simulink model "metro_queue"  (R2018b)
settings: Solver=VariableStepAuto  StartTime=0.0  StopTime=10.0  RelTol=1e-3
values from neighbouring files (symbols this model uses):
  entity_gen_period = 1.0 / current_mean_intensity    [metro_script.m]
undefined symbols (not defined in the file or in its folder): des
libraries: simeventslib x2
settings Model: Creator=kotvo  LastModifiedBy=marky

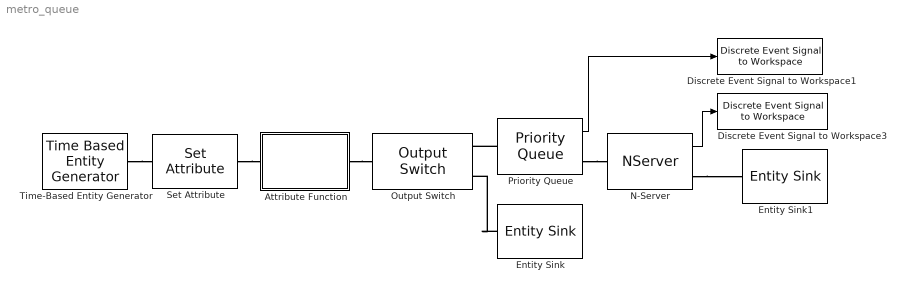
== system metro_queue ==
  Attribute Function : Subsystem  LoadFcn=des.afb.attributefunction_support(gcb,'LoadFcn');  StartFcn=des.afb.attributefunction_support(gcb,'StartFcn');  mask(Attribute Function){OutputNamePrefix=out_}
      mask prompts: OutputNamePrefix "Prefix name"
      settings: CopyFcn=des.afb.attributefunction_support(gcb,'CopyFcn');  OpenFcn=des.afb.attributefunction_support(gcb,'OpenFcn');  ErrorFcn=des.afb.error_redirect
      mask Help: slhelp(gcbh)
      mask Display: image(des_iconLoad('attribFunction.jpg'),'center');
  Discrete Event Signal to Workspace1 : simeventslib/SimEvents Sinks/Discrete Event Signal to Workspace  VariableName=average_wait  SaveFormat=Array  isMonitorOnly=off  isRecordIC=off
      settings: SourceProductName=SimEvents  SourceProductBaseCode=SE
  Discrete Event Signal to Workspace3 : simeventslib/SimEvents Sinks/Discrete Event Signal to Workspace  VariableName=processed_requests  SaveFormat=Array  isMonitorOnly=off  isRecordIC=off
      settings: SourceProductName=SimEvents  SourceProductBaseCode=SE
  Entity Sink : EntitySink
  Entity Sink1 : EntitySink
  N-Server : NServer  NumberOfServers=3  ServiceTime=2  StatNumberDeparted=on
  Output Switch : OutputSwitch  NumberOutputPorts=2
  Priority Queue : PriorityQueue  Capacity=current_queue_capacity  SortingAttributeName=priority  StatAverageWait=on
      settings: OutputPortMap=o2
  Set Attribute : SetAttribute  AttributeName=priority  EvaluatedAttributeValue={ 1}
  Time-Based Entity Generator : TimeBasedEntityGenerator  Distribution=Exponential  Period=entity_gen_period  Maximum=5  Mean=entity_gen_period
  wires:
  N-Server/1 -> Discrete Event Signal to Workspace3/1
  Priority Queue/1 -> Discrete Event Signal to Workspace1/1
  connections:
  Entity Sink/LConn1 -- Output Switch/RConn2
  Priority Queue/LConn1 -- Output Switch/RConn1
  N-Server/RConn1 -- Entity Sink1/LConn1
  Set Attribute/RConn1 -- Attribute Function/LConn1
  Attribute Function/RConn1 -- Output Switch/LConn1
  Priority Queue/RConn1 -- N-Server/LConn1
  Time-Based Entity Generator/RConn1 -- Set Attribute/LConn1

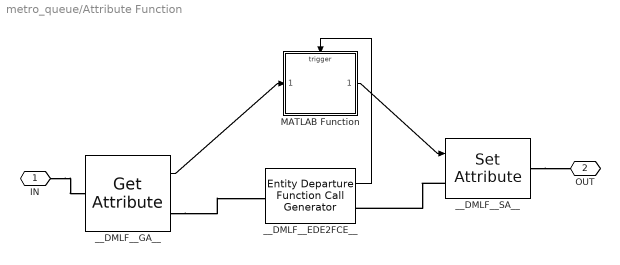
== system metro_queue/Attribute Function ==
  MATLAB Function : MATLAB Function  TreatAsAtomicUnit=on
  __DMLF__EDE2FCE__ : EntityDepartureFunctionCallGenerator  TimingFunctionCallF1=Before entity departure  IsInsideAFB=on
  __DMLF__GA__ : GetAttribute  AttributeName=priority  AttributeSendTiming=Before entity departure  EvaluatedDefaultAttributeValue={ []}  IsInsideAFB=on
      settings: OutputPortMap=o1
  __DMLF__SA__ : SetAttribute  AttributeName=priority  AttributeFrom=Signal port  EvaluatedAttributeValue={ []}  IsInsideAFB=on
  IN : PMIOPort  Side=Left
  OUT : PMIOPort  Port=2  Side=Right
  wires:
  __DMLF__EDE2FCE__/1 -> MATLAB Function/Trigger
  __DMLF__GA__/1 -> MATLAB Function/1(priority)
  MATLAB Function/1(out_priority) -> __DMLF__SA__/1
  connections:
  __DMLF__SA__/LConn1 -- __DMLF__EDE2FCE__/RConn1
  __DMLF__GA__/RConn1 -- __DMLF__EDE2FCE__/LConn1
  IN/RConn1 -- __DMLF__GA__/LConn1
  __DMLF__SA__/RConn1 -- OUT/RConn1

== matlab function metro_queue/Attribute Function/MATLAB Function ==
  data: priority input; out_priority output
  events: trigger input FUNCTION_CALL_EVENT
function out_priority  = fcn(priority)
%FCN    Access and modify attributes with MATLAB 
% 
% Input arguments must match the attribute names.
% Output arguments must be out_<AttributeName>,
% e.g., out_ServiceTime where ServiceTime is the attribute name.
% 
% The output attribute will be created if it is not present.
%
r = rand();
if r < 0.05
    out_priority = 2;
else
    out_priority = 1;
end
